simulink model "DynamicSpectrumAllocationDraft"  (R2024a)
settings: Solver=VariableStepAuto  StartTime=0.0  StopTime=10.0  RelTol=1e-3
settings Model: Creator=sampa  LastModifiedBy=sampa

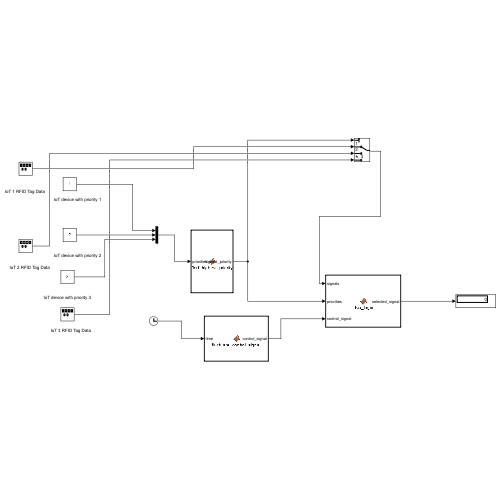
[thumbnail: Simulink's stored preview of the top-level diagram]
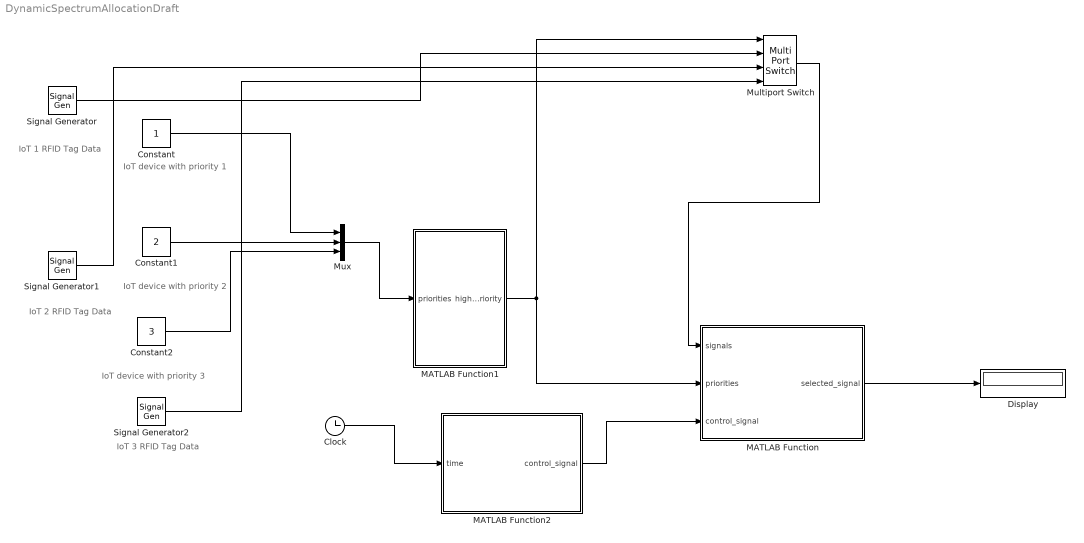
== system DynamicSpectrumAllocationDraft ==
  note: IoT device with priority 1
  note: IoT 1 RFID Tag Data
  note: IoT 2 RFID Tag Data
  note: IoT 3 RFID Tag Data
  note: IoT device with priority 2
  note: IoT device with priority 3
  Clock : Clock
  Constant : Constant
  Constant1 : Constant  Value=2
  Constant2 : Constant  Value=3
  Display : Display
      settings: Decimation=2
  MATLAB Function : MATLAB Function  TreatAsAtomicUnit=on
  MATLAB Function1 : MATLAB Function  TreatAsAtomicUnit=on
  MATLAB Function2 : MATLAB Function  TreatAsAtomicUnit=on
  Multiport Switch : MultiPortSwitch  DiagnosticForDefault=None  SaturateOnIntegerOverflow=off  InputSameDT=off
  Mux : Mux  Inputs=3
  Signal Generator : SignalGenerator  Amplitude=10  Frequency=65  Units=rad/sec
  Signal Generator1 : SignalGenerator  Amplitude=20  Frequency=65  Units=rad/sec
  Signal Generator2 : SignalGenerator  Amplitude=30  Frequency=65  Units=rad/sec
  wires:
  Signal Generator/1 -> Multiport Switch/2
  Signal Generator1/1 -> Multiport Switch/3
  Signal Generator2/1 -> Multiport Switch/4
  Multiport Switch/1 -> MATLAB Function/1(signals)
  Constant/1 -> Mux/1
  Constant1/1 -> Mux/2
  Constant2/1 -> Mux/3
  Mux/1 -> MATLAB Function1/1(priorities)
  MATLAB Function1/1(highest_priority) -> Multiport Switch/1, MATLAB Function/2(priorities)
  MATLAB Function/1(selected_signal) -> Display/1
  MATLAB Function2/1(control_signal) -> MATLAB Function/3(control_signal)
  Clock/1 -> MATLAB Function2/1(time)

== matlab function DynamicSpectrumAllocationDraft/MATLAB Function ==
  data: signals input; selected_signal output; priorities input; control_signal input
function selected_signal = dsa_logic(signals, priorities, control_signal)
    % Inputs:
    % signals       - a vector of signals from the IoT devices (1 x 3)
    % priorities    - a vector of priorities (1 x 3) where lower number means higher priority
    % control_signal - a scalar (1 = channel available, 0 = channel busy)

    % Initialize the output signal to 0 (no transmission by default)
    selected_signal = 0;

    % Check if the spectrum is available
    if control_signal == 1
        % Find the highest priority signal (smallest value in priorities)
        [~, highest_priority_index] = min(priorities);
        
        % Transmit the signal from the highest-priority device
        selected_signal = signals(highest_priority_index);
    else
        % If spectrum is busy (control_signal == 0), do not transmit anything
        selected_signal = 0;
    end
    disp(selected_signal)
end

== matlab function DynamicSpectrumAllocationDraft/MATLAB Function2 ==
  data: time input; control_signal output
function control_signal = fluctuate_control_signal(time)
    % Set the period of fluctuation
    period = 1;  % Time in seconds for one complete cycle
    % Calculate the control signal based on the current time
    if mod(floor(time), 2) == 0
        control_signal = int32(1);  % Set to 1 for even seconds
    else
        control_signal = int32(0);  % Set to 0 for odd seconds
    end
end

== matlab function DynamicSpectrumAllocationDraft/MATLAB Function1 ==
  data: priorities input; highest_priority output
function highest_priority = find_highest_priority(priorities)
    % Input:
    % priorities: A vector of priorities [priority1, priority2, priority3]
    
    % Initialize highest priority to zero
    highest_priority = 0;
    
    % Check for highest priority
    for i = 1:length(priorities)
        if priorities(i) > highest_priority
            highest_priority = priorities(i);
        end
    end
    highest_priority = 3;
end
